simulink model "que4"  (R2023a)
settings: Solver=VariableStepAuto  StartTime=0.0  StopTime=150  RelTol=1e-3
settings Model: Creator=sdz15  LastModifiedBy=Administrator
settings OptimizationCC: ReuseModelBlockBuffer=off

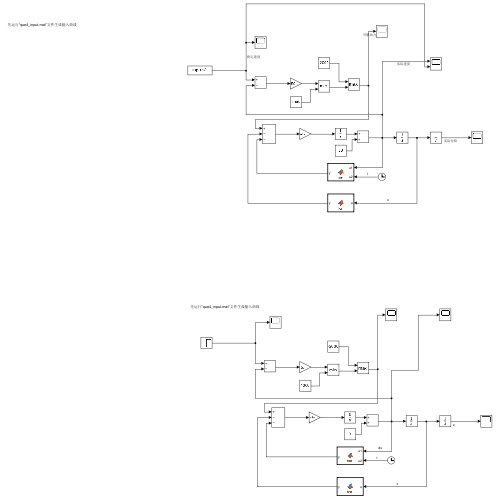
[thumbnail: Simulink's stored preview of the top-level diagram]
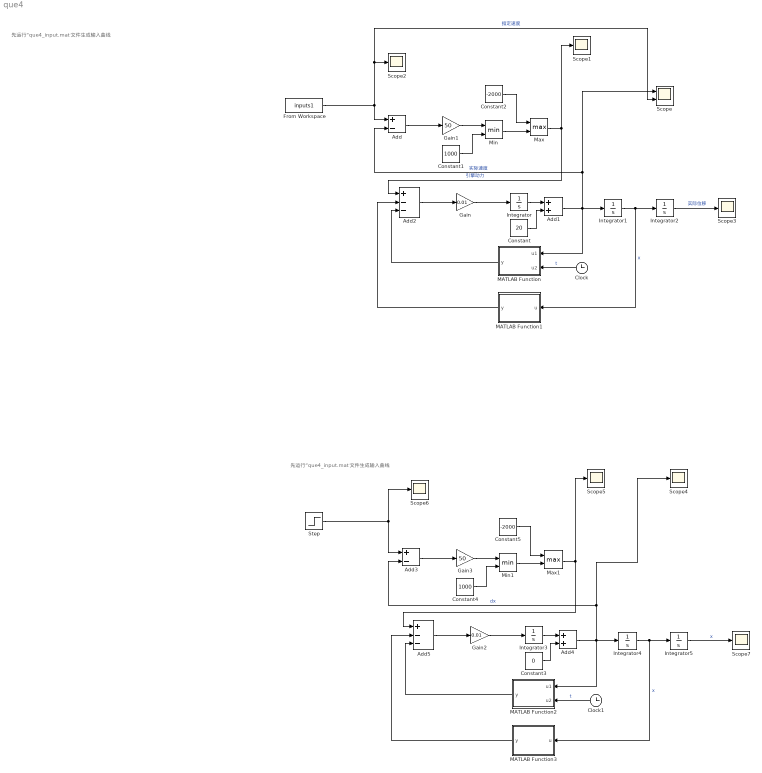
== system que4 ==
  note: 先运行“que4_input.mat”文件生成输入曲线
  note: 先运行“que4_input.mat”文件生成输入曲线
  Add : Sum  Inputs=+-
  Add1 : Sum
  Add2 : Sum  Inputs=+--
  Add3 : Sum  Inputs=+-
  Add4 : Sum
  Add5 : Sum  Inputs=+--
  Clock : Clock
  Clock1 : Clock
  Constant : Constant  Value=20
  Constant1 : Constant  Value=1000
  Constant2 : Constant  Value=-2000
  Constant3 : Constant  Value=0
  Constant4 : Constant  Value=1000
  Constant5 : Constant  Value=-2000
  From Workspace : FromWorkspace  VariableName=inputs1
  Gain : Gain  Gain=0.01
  Gain1 : Gain  Gain=50
  Gain2 : Gain  Gain=0.01
  Gain3 : Gain  Gain=50
  Integrator{,1..5} (6 alike) : Integrator
  MATLAB Function : MATLAB Function  TreatAsAtomicUnit=on
  MATLAB Function1 : MATLAB Function  TreatAsAtomicUnit=on
  MATLAB Function2 : MATLAB Function  TreatAsAtomicUnit=on
  MATLAB Function3 : MATLAB Function  TreatAsAtomicUnit=on
  Max : MinMax  Function=max  Inputs=2
  Max1 : MinMax  Function=max  Inputs=2
  Min : MinMax  Inputs=2
  Min1 : MinMax  Inputs=2
  Scope : Scope  NumInputPorts=2
  Scope{1..7} (7 alike) : Scope
  Step : Step  After=60  SampleTime=0
  wires:
  Integrator1/1 -> Integrator2/1, MATLAB Function1/1(u)  "x"
  MATLAB Function1/1(y) -> Add2/2
  From Workspace/1 -> Scope2/1, Scope/2, Add/1  "指定速度"
  Min/1 -> Max/2
  MATLAB Function/1(y) -> Add2/3
  Gain/1 -> Integrator/1
  Constant/1 -> Add1/2
  Add2/1 -> Gain/1
  Add1/1 -> Add/2, Scope/1, MATLAB Function/1(u1), Integrator1/1  "实际速度"
  Integrator/1 -> Add1/1
  Constant2/1 -> Max/1
  Clock/1 -> MATLAB Function/2(u2)  "t"
  Max/1 -> Add2/1, Scope1/1  "引擎动力"
  Constant1/1 -> Min/2
  Gain1/1 -> Min/1
  Add/1 -> Gain1/1
  Integrator2/1 -> Scope3/1  "实际位移"
  Min1/1 -> Max1/2
  Add3/1 -> Gain3/1
  Gain3/1 -> Min1/1
  Clock1/1 -> MATLAB Function2/2(u2)  "t"
  Constant5/1 -> Max1/1
  Integrator3/1 -> Add4/1
  MATLAB Function3/1(y) -> Add5/2
  Add4/1 -> Add3/2, Scope4/1, MATLAB Function2/1(u1), Integrator4/1  "dx"
  Constant4/1 -> Min1/2
  Gain2/1 -> Integrator3/1
  Max1/1 -> Add5/1, Scope5/1
  Add5/1 -> Gain2/1
  Integrator4/1 -> Integrator5/1, MATLAB Function3/1(u)  "x"
  Constant3/1 -> Add4/2
  Step/1 -> Add3/1, Scope6/1
  Integrator5/1 -> Scope7/1  "x"
  MATLAB Function2/1(y) -> Add5/3

== matlab function que4/MATLAB Function ==
  data: u1 input; y output; u2 input
function y = fcn(u1,u2)

y = 0.0001*((u1)+20*sin(0.01*(u2)))^2;
end

== matlab function que4/MATLAB Function2 ==
  data: u1 input; y output; u2 input
function y = fcn(u1,u2)

y = 0.0001*((u1)+20*sin(0.01*(u2)))^2;
end

== matlab function que4/MATLAB Function3 ==
  data: u input; y output
function y = fcn(u)

y = 30*sin(0.0001*(u));
end

== matlab function que4/MATLAB Function1 ==
  data: u input; y output
function y = fcn(u)

y = 30*sin(0.0001*(u));
end
